simulink model "Shaft_2_2"  (R2023a)
settings: Solver=FixedStepAuto  StartTime=0.0  StopTime=2000.0  FixedStep=0.01  RelTol=1e-3
values from neighbouring files (symbols this model uses):
  shaft2_F2 = - moments(2).F * shaft2_l3 / (shaft2_l3 - shaft2_l2)    [Shaft_data.m]
  shaft2_F3 = moments(2).F * shaft2_l2 / (shaft2_l3 - shaft2_l2)    [Shaft_data.m]
  shaft2_l2 = 500    [Shaft_data.m]
  shaft2_l3 = 750    [Shaft_data.m]
undefined symbols (not defined in the file or in its folder): moments
settings Model: Creator=User  LastModifiedBy=User

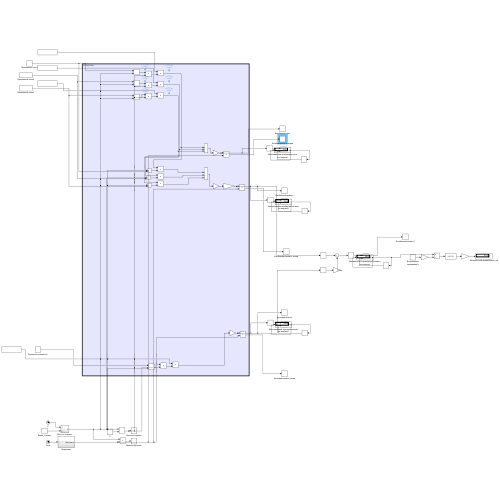
[thumbnail: Simulink's stored preview of the top-level diagram]
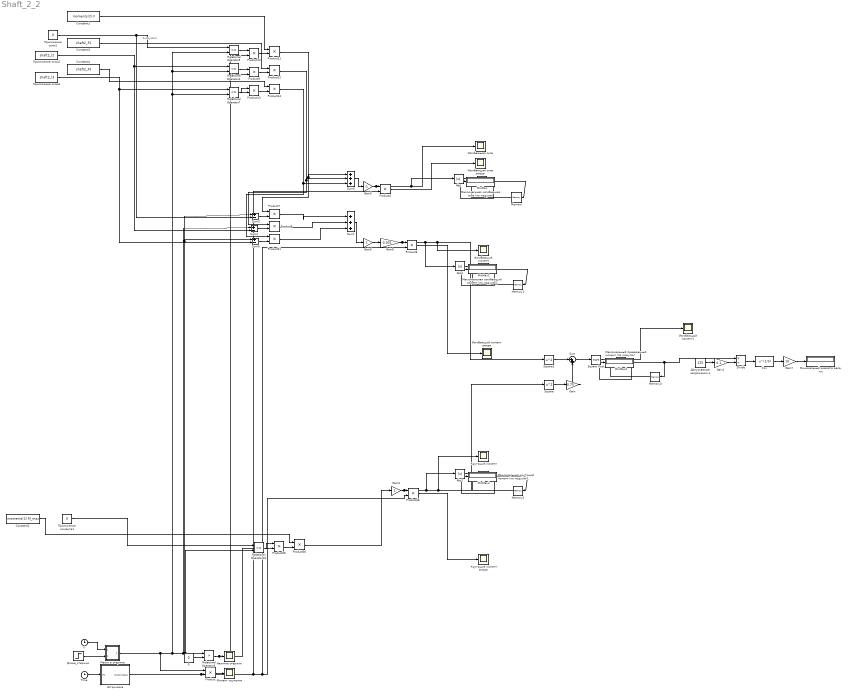
== system Shaft_2_2 ==
  note: Subsystem
  0 : Constant  Value=0
  Abs : Abs  SaturateOnIntegerOverflow=off
  Abs1 : Abs  SaturateOnIntegerOverflow=off
  Abs2 : Abs  SaturateOnIntegerOverflow=off
  Constant1 : Constant  Value=moments(2).F
  Constant2 : Constant  Value=moments(2).M_max
  Constant3 : Constant  Value=shaft2_F2
  Constant4 : Constant  Value=shaft2_F3
  Divide : Product  Inputs=*/
  Fcn : Fcn  Expr=u^(1/3)
  Gain : Gain  Gain=0.75
  Gain1 : Gain  Gain=0.1
  Gain2 : Gain
  Gain5 : Gain  Gain=-1
  Gain6 : Gain
  Gain7 : Gain  Gain=10
  Gain8 : Gain  Gain=0.001
  Memory{,1..3} (4 alike) : Memory  InitialCondition=-10000
  MinMax{,1..3} (4 alike) : MinMax  Function=max  Inputs=2
  Product{,4,6..14,21,35..36,46} (15 alike) : Product
  Relational Operator{4..5,7,15} (4 alike) : RelationalOperator  Operator=<=  OutDataTypeStr=boolean  RndMeth=Simplest  InputSameDT=off
  Relational Operator6 : RelationalOperator  Operator=>  OutDataTypeStr=boolean  RndMeth=Simplest  InputSameDT=off
  Square : Math  Operator=square
  Square Root : Sqrt
  Square1 : Math  Operator=square
  Sum : Sum  Inputs=|++
  Sum1 : Sum  Inputs=|+++
  Sum2 : Sum  Inputs=|+-
  Sum3 : Sum  Inputs=|+-
  Sum5 : Sum  Inputs=|+-
  Sum9 : Sum  Inputs=|+++
  Time : Clock
      settings: Decimation=15
  X : Clock
      settings: Decimation=15
  Длина_стержня : Step  Time=1500  After=1000  SampleTime=0
  Допускаемые напряжения σ : Constant  Value=125
  Изгибающая сила : Scope
  Изгибающая сила эпюра : Scope
  Изгибающий момент : Scope
  Изгибающий момент эпюра : Scope
  Изгибающий момент1 : Scope
  Крутящий момент : Scope
  Крутящий момент эпюра : Scope
  Максимальная изгибающая сила (по модулю) : Display
  Максимальная изгибающий момент (по модулю)1 : Display
  Максимальный крутящий момент (по модулю)1 : Display
  Максимальный приведенный момент (по модулю) : Display
  Место в стержне : Subsystem
  "Минимальный диаметр вала, мм" : Display
  Момент кручения : Scope
  Наличие стержня : Scope
  Приложение момента1 : Constant  Value=0
  Приложение силы1 : Constant  Value=0
  Приложение силы2 : Constant  Value=shaft2_l2
  Приложение силы3 : Constant  Value=shaft2_l3
  Штриховка : Subsystem
  wires:
  Fcn/1 -> Gain7/1
  Abs2/1 -> MinMax2/1
  Допускаемые напряжения σ/1 -> Gain1/1
  Abs1/1 -> MinMax1/1
  MinMax3/1 -> Divide/1, Memory3/1, Максимальный приведенный момент (по модулю)/1
  Gain1/1 -> Divide/2
  Memory2/1 -> MinMax2/2
  Product/1 -> Момент кручения/1
  Divide/1 -> Fcn/1
  Square/1 -> Gain/1
  Sum/1 -> Square Root/1
  Memory3/1 -> MinMax3/2
  MinMax2/1 -> Максимальный крутящий момент (по модулю)1/1, Memory2/1
  Square Root/1 -> Изгибающий момент1/1, MinMax3/1
  Abs/1 -> MinMax/1
  X/1 -> Место в стержне/1(In1)
  Memory1/1 -> MinMax1/2
  Time/1 -> Штриховка/1(In1)
  Длина_стержня/1 -> Место в стержне/2(In2)
  MinMax/1 -> Максимальная изгибающая сила (по модулю)/1, Memory/1
  Gain/1 -> Sum/2
  Square1/1 -> Sum/1
  0/1 -> Relational Operator6/2
  MinMax1/1 -> Максимальная изгибающий момент (по модулю)1/1, Memory1/1
  Memory/1 -> MinMax/2
  Gain7/1 -> "Минимальный диаметр вала, мм"/1
  Gain8/1 -> Square1/1, Изгибающий момент/1, Abs1/1, Product6/1
  Gain2/1 -> Square/1, Крутящий момент/1, Abs2/1, Product46/1
  Gain5/1 -> Abs/1, Изгибающая сила/1, Product4/1
  Product4/1 -> Изгибающая сила эпюра/1
  Product6/1 -> Изгибающий момент эпюра/1
  Product46/1 -> Крутящий момент эпюра/1
  Product36/1 -> Gain2/1
  Product35/1 -> Product36/2
  Product21/1 -> Sum1/3
  Relational Operator7/1 -> Product13/1
  Product9/1 -> Product12/2
  Product11/1 -> Product7/1, Sum9/1
  Product12/1 -> Product8/1, Sum9/2
  Gain6/1 -> Gain8/1
  Relational Operator4/1 -> Product9/1
  Relational Operator15/1 -> Product35/1
  Sum1/1 -> Gain6/1
  Product8/1 -> Sum1/2
  Sum5/1 -> Product21/2
  Product14/1 -> Product21/1, Sum9/3
  Sum2/1 -> Product8/2
  Relational Operator6/1 -> Product10/2, Product9/2, Product13/2, Product35/2, Наличие стержня/1
  Product7/1 -> Sum1/1
  Sum9/1 -> Gain5/1
  Product13/1 -> Product14/2
  Relational Operator5/1 -> Product10/1
  Product10/1 -> Product11/2
  Штриховка/1(Штриховка) -> Product46/2, Product6/2, Product4/2, Product/2
  Место в стержне/1(Out1) -> Relational Operator6/1, Relational Operator15/2, Sum3/1, Sum5/1, Sum2/1, Relational Operator5/2, Relational Operator4/2, Relational Operator7/2, Product/1
  Sum3/1 -> Product7/2
  Приложение силы1/1 -> Sum3/2, Relational Operator5/1
  Приложение силы2/1 -> Sum2/2, Relational Operator4/1
  Приложение силы3/1 -> Sum5/2, Relational Operator7/1
  Constant1/1 -> Product11/1
  Приложение момента1/1 -> Relational Operator15/1
  Constant2/1 -> Product36/1
  Constant3/1 -> Product12/1
  Constant4/1 -> Product14/1

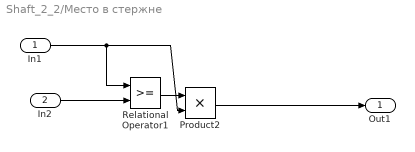
== system Shaft_2_2/Место в стержне ==
  In1 : Inport
  In2 : Inport  Port=2
  Product2 : Product
  Relational Operator1 : RelationalOperator  OutDataTypeStr=boolean  RndMeth=Simplest  InputSameDT=off
  Out1 : Outport
  wires:
  Relational Operator1/1 -> Product2/1
  Product2/1 -> Out1/1
  In2/1 -> Relational Operator1/2
  In1/1 -> Product2/2, Relational Operator1/1

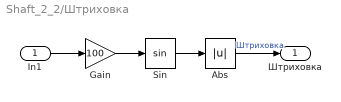
== system Shaft_2_2/Штриховка ==
  In1 : Inport
  Abs : Abs  SaturateOnIntegerOverflow=off
  Gain : Gain  Gain=100
  Sin : Trigonometry
  Штриховка : Outport
  wires:
  Sin/1 -> Abs/1
  In1/1 -> Gain/1
  Gain/1 -> Sin/1
  Abs/1 -> Штриховка/1  "Штриховка"
